simulink model "ej2_1"  (R2023a)
settings: Solver=VariableStepAuto  StartTime=0.0  StopTime=30.0  RelTol=1e-3
values from neighbouring files (symbols this model uses):
  x0 = [4; 1]    [ej2_1_script.m]
undefined symbols (not defined in the file or in its folder): a, b, c, d
settings Model: Creator=erwinplanck  LastModifiedBy=erwinplanck

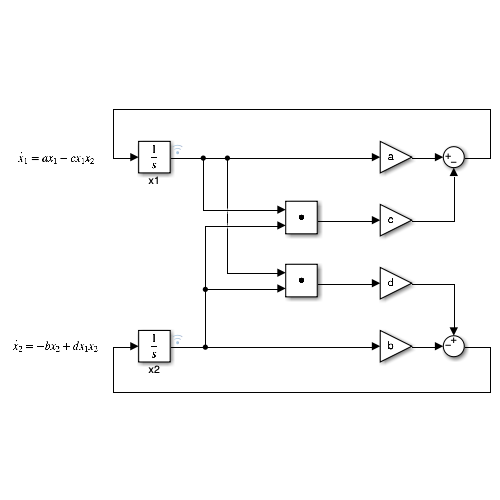
[thumbnail: Simulink's stored preview of the top-level diagram]
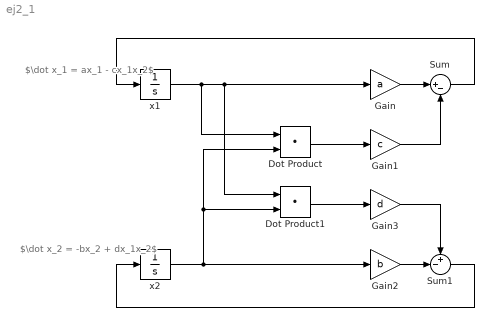
== system ej2_1 ==
  note: $\dot x_1 = ax_1 - cx_1x_2$
  note: $\dot x_2 = -bx_2 + dx_1x_2$
  Dot Product : DotProduct  OutDataTypeStr=Inherit: Inherit via internal rule
  Dot Product1 : DotProduct  OutDataTypeStr=Inherit: Inherit via internal rule
  Gain : Gain  Gain=a
  Gain1 : Gain  Gain=c
  Gain2 : Gain  Gain=b
  Gain3 : Gain  Gain=d
  Sum : Sum  Inputs=|+-
  Sum1 : Sum  Inputs=+-|
  x1 : Integrator  InitialCondition=x0(1, 1)
  x2 : Integrator  InitialCondition=x0(2, 1)
  wires:
  x1/1 -> Dot Product/1, Dot Product1/1, Gain/1
  x2/1 -> Gain2/1, Dot Product1/2, Dot Product/2
  Dot Product/1 -> Gain1/1
  Gain/1 -> Sum/1
  Gain1/1 -> Sum/2
  Sum/1 -> x1/1
  Dot Product1/1 -> Gain3/1
  Gain2/1 -> Sum1/2
  Gain3/1 -> Sum1/1
  Sum1/1 -> x2/1
